simulink model "Plantnl"  (Simulink 7.0)
settings: Solver=ode45  SolverMode=SingleTasking  StartTime=0.0  StopTime=100  RelTol=1e-3  AbsTol=1e-6
undefined symbols (not defined in the file or in its folder): Conduction, InputFlux, M_inv, Radiation, ScaleTemp
settings Model: Creator=abbas  LastModifiedBy=abbas
settings DataIOCC: LimitDataPoints=off
settings OptimizationCC: BlockReduction=off  BooleanDataType=off  InlineInvariantSignals=on
settings DebuggingCC: SaveWithParameterizedLinksMsg=none  SignalResolutionControl=TryResolveAllWithWarning  SolverPrmCheckMsg=none  MultiTaskDSMMsg=warning  MultiTaskCondExecSysMsg=none  StrictBusMsg=None
settings HardwareCC: TargetUnknown=on
settings RTWCC: IncludeERTFirstTime=on
settings GRTTargetCC: TargetFcnLib=ansi_tfl_tmw.mat  ModelReferenceCompliant=off  CompOptLevelCompliant=off  MatFileLogging=off

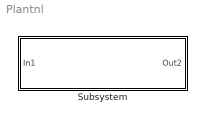
== system Plantnl ==
  Subsystem : Subsystem

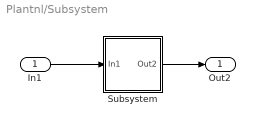
== system Plantnl/Subsystem ==
  In1 : Inport  OutDataType=sfix(16)  OutScaling=2^0
  Subsystem : Subsystem
  Out2 : Outport  OutDataType=sfix(16)  OutScaling=2^0
  wires:
  In1/1 -> Subsystem/1(In1)
  Subsystem/1(Out2) -> Out2/1

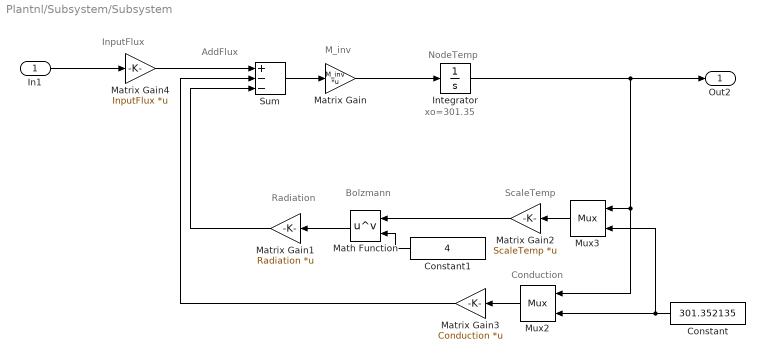
== system Plantnl/Subsystem/Subsystem ==
  note: InputFlux
  note: AddFlux
  note: M_inv
  note: NodeTemp
  note: xo=301.35
  note: Radiation
  note: ScaleTemp
  note: Conduction
  note: Bolzmann
  In1 : Inport  OutDataType=sfix(16)  OutScaling=2^0
  Constant : Constant  Orientation=left  Value=301.352135  OutDataType=sfix(16)  OutScaling=2^0
  Constant1 : Constant  Orientation=left  Value=4  OutDataType=sfix(16)  OutScaling=2^0
  Integrator : Integrator  InitialCondition=301.3521350999999
  Math Function : Math  Orientation=left  Operator=pow  OutDataType=sfix(16)  OutScaling=2^0  SaturateOnIntegerOverflow=on
  Matrix Gain : Gain  Gain=M_inv  Multiplication=Matrix(K*u)  ParameterDataType=sfix(16)  ParameterScaling=2^0  OutDataType=sfix(16)  OutScaling=2^0  SaturateOnIntegerOverflow=on
  Matrix Gain1 : Gain  Orientation=left  Gain=Radiation  Multiplication=Matrix(K*u)  ParameterDataType=sfix(16)  ParameterScaling=2^0  OutDataType=sfix(16)  OutScaling=2^0  SaturateOnIntegerOverflow=on
  Matrix Gain2 : Gain  Orientation=left  Gain=ScaleTemp  Multiplication=Matrix(K*u)  ParameterDataType=sfix(16)  ParameterScaling=2^0  OutDataType=sfix(16)  OutScaling=2^0  SaturateOnIntegerOverflow=on
  Matrix Gain3 : Gain  Orientation=left  Gain=Conduction  Multiplication=Matrix(K*u)  ParameterDataType=sfix(16)  ParameterScaling=2^0  OutDataType=sfix(16)  OutScaling=2^0  SaturateOnIntegerOverflow=on
  Matrix Gain4 : Gain  Gain=InputFlux  Multiplication=Matrix(K*u)  ParameterDataType=sfix(16)  ParameterScaling=2^0  OutDataType=sfix(16)  OutScaling=2^0  SaturateOnIntegerOverflow=on
  Mux2 : Mux  Orientation=left  Inputs=2
  Mux3 : Mux  Orientation=left  Inputs=2
  Sum : Sum  Inputs=+--  OutDataType=sfix(16)  OutScaling=2^0  SaturateOnIntegerOverflow=on  InputSameDT=on
  Out2 : Outport  OutDataType=sfix(16)  OutScaling=2^0
  wires:
  Matrix Gain4/1 -> Sum/1
  Sum/1 -> Matrix Gain/1
  Matrix Gain/1 -> Integrator/1
  Integrator/1 -> Mux2/1, Mux3/1, Out2/1
  Mux3/1 -> Matrix Gain2/1
  Mux2/1 -> Matrix Gain3/1
  Matrix Gain3/1 -> Sum/2
  Constant/1 -> Mux2/2, Mux3/2
  Matrix Gain1/1 -> Sum/3
  Math Function/1 -> Matrix Gain1/1
  Matrix Gain2/1 -> Math Function/1
  Constant1/1 -> Math Function/2
  In1/1 -> Matrix Gain4/1
